simulink subsystem "PieroModel"  (R2023b)
settings: Solver=VariableStepAuto  StartTime=0.0  StopTime=10.0  RelTol=1e-3
settings Model: Creator=chaya  LastModifiedBy=chaya

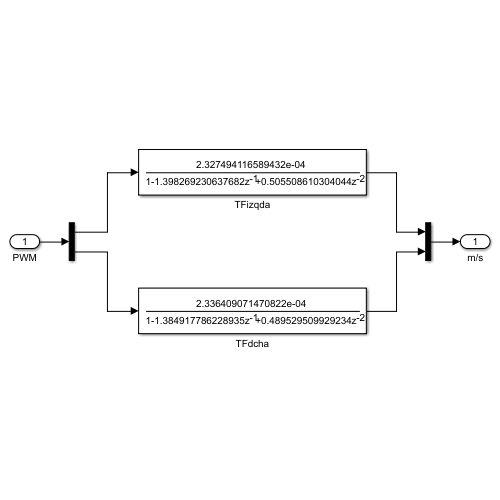
[thumbnail: Simulink's stored preview of the top-level diagram]
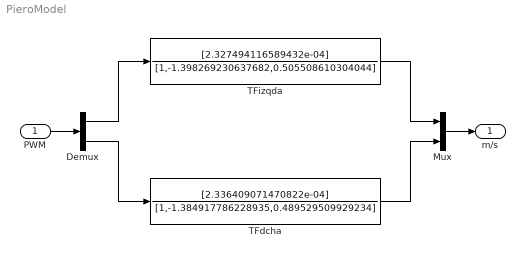
== system PieroModel ==
  PWM : Inport
  Demux : Demux  Outputs=2
  Mux : Mux  Inputs=2
  TFdcha : DiscreteFilter  Numerator=[2.336409071470822e-04]  Denominator=[1,-1.384917786228935,0.489529509929234]
  TFizqda : DiscreteFilter  Numerator=[2.327494116589432e-04]  Denominator=[1,-1.398269230637682,0.505508610304044]
  m/s : Outport
  wires:
  Mux/1 -> m/s/1
  PWM/1 -> Demux/1
  Demux/1 -> TFizqda/1
  TFizqda/1 -> Mux/1
  Demux/2 -> TFdcha/1
  TFdcha/1 -> Mux/2
